simulink library "AEMS_Standard_Library"  (R2016b)
(part 7 of 39)

      |         maskobj_param(3).Enabled = 'on';
      |         switch(Outputs_From_get_param)
      |             case '1'
      |                 Non=4;
      |             case '2'
      |                 Non=5;
      |             case '3'
      |                 Non=6;
      |              case '4'
      |                  Non=7;
      |              case '6'
      |                  Non=9;
      |              case '8'
      |                  Non=11;
      |         end
      |     else
      |         maskobj_param(3).Visible = 'off';
      |         maskobj_param(3).Enabled = 'off';
      |         Non=4;
      |     end
      | for i=4:Non
      |     maskobj_param(i).Visible = 'on';
      |     maskobj_param(i).Enabled = 'on';
      | end
      | for i=Non+1:11
      |     maskobj_param(i).Visible = 'off';
      |     maskobj_param(i).Enabled = 'off';
      | end
      | clear maskobj_param;
      | clear maskobj;
      mask TypeOptions Dim_num: 1 | 2 | 3 | 4 | 6 | 8
      mask Callback Dim_num:
      | Outputs_From_get_param = get_param(gcb,'Dim_num');
      | Specificchoice_get_param = get_param(gcb,'Specificchoix');
      | maskobj = Simulink.Mask.get(gcbh);
      | maskobj_param = maskobj.Parameters;
      |     if strcmpi(Specificchoice_get_param,'on')
      |        Non=4;
      |         maskobj_param(3).Visible = 'on';
      |         maskobj_param(3).Enabled = 'on';
      |         switch(Outputs_From_get_param)
      |             case '1'
      |                 Non=4;
      |             case '2'
      |                 Non=5;
      |             case '3'
      |                 Non=6;
      |              case '4'
      |                  Non=7;
      |              case '6'
      |                  Non=9;
      |              case '8'
      |                  Non=11;
      |         end
      |     else
      |         maskobj_param(3).Visible = 'off';
      |         maskobj_param(3).Enabled = 'off';
      |         Non=4;
      |     end
      | for i=4:Non
      |     maskobj_param(i).Visible = 'on';
      |     maskobj_param(i).Enabled = 'on';
      | end
      | for i=Non+1:11
      |     maskobj_param(i).Visible = 'off';
      |     maskobj_param(i).Enabled = 'off';
      | end
      | clear maskobj_param;
      | clear maskobj;
      mask TypeOptions DemDebounceBehavior1: DEM_DEBOUNCE_FREEZE (0) | DEM_DEBOUNCE_RESET (1)
      mask TypeOptions DemDebounceBehavior2: DEM_DEBOUNCE_FREEZE (0) | DEM_DEBOUNCE_RESET (1)
      mask TypeOptions DemDebounceBehavior3: DEM_DEBOUNCE_FREEZE (0) | DEM_DEBOUNCE_RESET (1)
      mask TypeOptions DemDebounceBehavior4: DEM_DEBOUNCE_FREEZE (0) | DEM_DEBOUNCE_RESET (1)
      mask TypeOptions DemDebounceBehavior5: DEM_DEBOUNCE_FREEZE (0) | DEM_DEBOUNCE_RESET (1)
      mask TypeOptions DemDebounceBehavior6: DEM_DEBOUNCE_FREEZE (0) | DEM_DEBOUNCE_RESET (1)
      mask TypeOptions DemDebounceBehavior7: DEM_DEBOUNCE_FREEZE (0) | DEM_DEBOUNCE_RESET (1)
      mask TypeOptions DemDebounceBehavior8: DEM_DEBOUNCE_FREEZE (0) | DEM_DEBOUNCE_RESET (1)
      mask TypeOptions sampletime: 0.001 | 0.002 | 0.004 | 0.01 | 0.02 | 0.1
  AEMS_DEM_TIME_BASED_DEBOUNCE_THRSHOLD_DYN : Subsystem  Tag=[LIB]  Description=This subsystem is interface for self diagnosis standard calculated from similar condition and NG judgment.  mask(AEMS_DEM_TIME_BASED_DEBOUNCE_THRSHOLD_DYN){eventid=Dem_EventId_Device_Faulttype, Specificchoix=off, Dim_num=1, DemDebounceBehavior1=DEM_DEBOUNCE_FREEZE (0), DemDebounceBehavior2=DEM_DEBOUNCE_RESET (1), DemDebounceBehavior3=DEM_DEBOUNCE_FREEZE (0), DemDebounceBehavior4=DEM_DEBOUNCE_FREEZE (0), DemDebounceBehavior5=DEM_DEBOUNCE_RESET (1), DemDebounceBehavior6=DEM_DEBOUNCE_RESET (1), DemDebounceBehavior7=DEM_DEBOUNCE_FREEZE (0), DemDebounceBehavior8=DEM_DEBOUNCE_FREEZE (0), DemTimeBypassFailure=Cbx_dem_byp_fail_Device_Faulttype, sampletime=0.01, ToDataStoreMemory=off}
      mask prompts: eventid "Identifier of a diagnostic event (EventId)"; Specificchoix "Specific case used only for Nissan cases"; Dim_num "Time_Based_Debounce_Dimension"; DemDebounceBehavior1 "Dem Debounce Behavior 1"; DemDebounceBehavior2 "Dem Debounce Behavior 2"; DemDebounceBehavior3 "Dem Debounce Behavior 3"; DemDebounceBehavior4 "Dem Debounce Behavior 4"; DemDebounceBehavior5 "Dem Debounce Behavior 5"; DemDebounceBehavior6 "Dem Debounce Behavior 6"; DemDebounceBehavior7 "Dem Debounce Behavior 7"; DemDebounceBehavior8 "Dem Debounce Behavior 8"; DemTimeBypassFailure "Dem Debounce Time Bypass Failure"; sampletime "Sample Time"; ToDataStoreMemory "Write Output To Data Store Memory"
      mask help:
      | It  transmit the status Failed or Passed to the DEM. Accordingly,
      | some bits of the UDS DTC status byte changes synchronously or
      | asynchronously according to the configuration.
      |
      | -INPUTS-
      | conditionfulfilled: specifies whether the storage condition assigned
      | to the StorageConditionId is fulfilled
      | prefailed: Monitor reports nonqualified test result pre-failed
      | prepassed: Monitor reports nonqualified test result pre-passed
      | ClearDataRequest:Clears the Data Request value
      | reseteventdebounce: Freeze or reset the internal debounce timer.
      | failedthreshold: Defines the time out duration for "Event Failed" qualification.
      | passedthreshold: Defines the time out duration for "Event Passed" qualification.
      |
      | -OUTPUTS-
      | debouncevalue_for_failed: Value of debounce when an event failed
      | debouncevalue_for_passed: Value of debounce when an event passed
      | failed: Diagnostic monitor reports an event failed
      | passed: Diagnostic monitor reports an event passed
      |
      | -PARAMETERS-
      | EventId: Internal identifier of a diagnostic event. 0 is not a valid value.
      | Debounce Behavior: The event debounce counter will be frozen or reset
      | (0 for FREEZE and 1 for RESET)
      mask init:
      | lib_path = gcb;
      | Current_Child_Lib_Path = find_system(lib_path,'LookUnderMasks','all','FollowLinks','on','Name','AEMS_DEM_TIME_BASED_DEBOUNCE_THRSHOLD_DYN_D');
      | Attribute_Format_String_Part1 = '%<MaskType>\n EventId : %<eventid> \n Specific case used only for Nissan cases = %<Specificchoix> ';
      | Attribute_Format_String_Part2 = '';
      | if strcmpi(Specificchoix,'off')
      |     Dim_num = '1';
      | else
      |     Attribute_Format_String_Part2 = '\n Time_Based_Debounce_Dimention = %<Dim_num> ';
      | end
      | dim_block = ['AEMS_DEM_TIME_BASED_DEBOUNCE_THRSHOLD_DYN_' Dim_num 'D'];
      | 
      | rep_block = ['AEMS_Standard_Library/SUB/',dim_block];
      | if ismember(get_param(Current_Child_Lib_Path,'MaskType'),{dim_block})
      | else
      |     replace_block(lib_path,'FollowLinks','on','Name','AEMS_DEM_TIME_BASED_DEBOUNCE_THRSHOLD_DYN_D',rep_block,'noprompt');
      | end
      | 
      | Attribute_Format_String_Part3='';
      | for i=1:str2num(Dim_num)
      |     Attribute_Format_String_Part3=[Attribute_Format_String_Part3,'\n Dem Debounce Behavior ',num2str(i),' = %<DemDebounceBehavior',num2str(i),'>'];
      |     set_param([Current_Child_Lib_Path{:}],['DemDebounceBehavior',num2str(i)],get_param(lib_path,['DemDebounceBehavior',num2str(i)]));
      | end
      | 
      | sampletime_tmp = get_param(lib_path,'sampletime');
      | DemTimeBypassFailure_tmp = get_param(lib_path,'DemTimeBypassFailure');
      | 
      | set_param([Current_Child_Lib_Path{:}],'eventid',eventid);
      | set_param([Current_Child_Lib_Path{:}],'Sample_Time',sampletime_tmp);
      | set_param([Current_Child_Lib_Path{:}],'DemTimeBypassFailure',DemTimeBypassFailure_tmp);
      | 
      | %If To DataStoreMemory is enabled...
      | if strcmpi(ToDataStoreMemory,'on') && isempty(find_system(lib_path,'LookUnderMasks','all','FollowLinks','on','Name','AEMS_SRFLIPFLOP'))
      |     add_block('AEMS_Standard_Library/FLAG/AEMS_SRFLIPFLOP',[lib_path,'/AEMS_SRFLIPFLOP'],'Position',[930 254 1015 376]);
      |     add_block('simulink/Signal Attributes/Data Type Conversion',[lib_path,'/Data Type Conversion'],'Position',[1060 303 1115 327],'ShowName','off')
      |     add_block('simulink/Signal Routing/Data Store Write',[lib_path,'/Data Store Write'],'Position',[1160 302 1385 328],'ShowName','off');
      |     add_line(lib_path,'AEMS_DEM_TIME_BASED_DEBOUNCE_THRSHOLD_DYN_D/3','AEMS_SRFLIPFLOP/1','AutoRouting','on');
      |     add_line(lib_path,'AEMS_DEM_TIME_BASED_DEBOUNCE_THRSHOLD_DYN_D/4','AEMS_SRFLIPFLOP/2','AutoRouting','on');
      |     add_line(lib_path,'AEMS_SRFLIPFLOP/1','Data Type Conversion/1');
      |     add_line(lib_path,'Data Type Conversion/1','Data Store Write/1');
      | elseif strcmpi(ToDataStoreMemory,'off') && ~isempty(find_system(lib_path,'LookUnderMasks','all','FollowLinks','on','Name','AEMS_SRFLIPFLOP'))
      |     delete_block([lib_path,'/AEMS_SRFLIPFLOP']);
      |     delete_block([lib_path,'/Data Type Conversion']);
      |     delete_block([lib_path,'/Data Store Write']);
      |     delete_line(find_system(lib_path,'FollowLinks','on','FindAll','on','LookUnderMasks','on','Type','line','Connected','off'));
      | end
      | 
      | if strcmpi(ToDataStoreMemory,'on')
      |     %Get Task Rate of this block.(As per AEMS arch, all the blks shall be
      |     %kept under the runnable. The Runnable name will ncontain the sample
      |     %time suffix. From where we can get it.
      |     model_type_pos = strsplit(lib_path,'/');%to split all the layer paths in order to get the runnable path
      |     runnable_path = [bdroot '/' model_type_pos{2}];%to get the runnable or AIPCALL path
      |     trg_port_name = get_param(find_system(runnable_path,'BlockType','TriggerPort'),'Name');%to get the function call trigger name
      |     TaskRate = '';%the raster suffix is stored in the parameter
      |     
      |     if ~isempty(trg_port_name)
      |         trg_port_name_spltd = strsplit(trg_port_name{1},'_');%splitting is done in order to get the raster and its type(Sched or Event)
      |         
      |         % checking for rasters of type Sched or Event especially occuring in
      |         % runnables
      |         if ~isempty(regexp(trg_port_name_spltd{1},'^Sched|^Event','once'))
      |             TaskRate = ['_' regexprep(trg_port_name_spltd{1},'Sched|Event','','once')];
      |             
      |             %checking if the raster is dcmcb and this is applicable only for
      |             %APICALL
      |         elseif ~isempty(regexp([trg_port_name_spltd{1} '_' trg_port_name_spltd{2} '_' ],'^DataServices_DCM_|^RoutineServices_DCM_','once'))||...
      |                 ~isempty(regexp(trg_port_name_spltd{1},'^Dcm$','once'))
      |             TaskRate = '_dcmcb';
      |             
      |             %checking if this block is used under the function call trigger
      |             %starting with "Com" and then giving an error message
      |             %this is applicable only for APICALL
      |         elseif ~isempty(regexp(trg_port_name_spltd{1},'^Com$','once'))
      |             msg = sprintf(['\n','The FIM block "' lib_path '" should not be present within APICALLs having function call trigger as "Com"']);
      |             errordlg(msg);
      |             return;
      |         end
      |     end
      |     DataStoreName = [eventid,TaskRate];
      |     set_param([lib_path,'/Data Store Write'],'DataStoreName',DataStoreName);
      | end
      | 
      | Attribute_Format_String_Part5 = '\n Write Output To Data Store Memory := %<ToDataStoreMemory>';
      | 
      | 
      | Attribute_Format_String_Part4='\nDem Debounce Time Bypass Failure = %<DemTimeBypassFailure>\nSample Time = %<sampletime>';
      | Attribute_Format_String = [Attribute_Format_String_Part1,Attribute_Format_String_Part2,Attribute_Format_String_Part3,Attribute_Format_String_Part4, Attribute_Format_String_Part5];
      | 
      | set_param(lib_path,'AttributesFormatString',Attribute_Format_String);
      settings: AttributesFormatString=%<MaskType>\n EventId : %<eventid> \n Specific case used only for Nissan cases = %<Specificchoix> \n Dem Debounce Behavior 1 = %<DemDebounceBehavior1>\nDem Debounce Time Bypass Failure = %<DemTimeBypassFailure>\nSample Time = %<sampletime>\n Write Output To Data Store Memory := %<ToDataStoreMemory>
      mask Help:
      | eval('path_lib=fileparts(which(''AEMS_Standard_Library''));');
      | doc_path = [path_lib '\help\AEMS_DEM_TIME_BASED_DEBOUNCE_THRSHOLD_DYN.pdf'];
      | eval('open(doc_path)');
      mask Callback eventid:
      | lib_path=gcb;
      | EventID=get_param(lib_path,'eventid');
      | Splitname=regexp(EventID,'_','all');
      | EventID_Name=extractAfter(EventID,EventID(1:Splitname(2)));
      | BypassFailure=strcat('Cbx_dem_byp_fail_',EventID_Name);
      | set_param(lib_path,'DemTimeBypassFailure',BypassFailure);
      | ToDataStoreMemory = get_param(lib_path,'ToDataStoreMemory');
      | 
      | if strcmpi(ToDataStoreMemory,'on')
      | model_type_pos = strsplit(lib_path,'/');%to split all the layer paths in order to get the runnable path
      | runnable_path = [bdroot '/' model_type_pos{2}];%to get the runnable or AIPCALL path
      | trg_port_name = get_param(find_system(runnable_path,'BlockType','TriggerPort'),'Name');%to get the function call trigger name
      | TaskRate = '';%the raster suffix is stored in the parameter
      | 
      | if ~isempty(trg_port_name)
      |     trg_port_name_spltd = strsplit(trg_port_name{1},'_');%splitting is done in order to get the raster and its type(Sched or Event)
      | 
      |     % checking for rasters of type Sched or Event especially occuring in
      |     % runnables
      |     if ~isempty(regexp(trg_port_name_spltd{1},'^Sched\d+(ms|s)$|^Event+(sync|knock|comc|coml|dcmcb)$','once'))
      |         TaskRate = ['_' regexp(trg_port_name_spltd{1},'\d+(ms|s)$|sync$|knock$|comc$|coml$|dcmcb$','match','once')];
      | 
      |     %checking if the raster is dcmcb and this is applicable only for
      |     %APICALL
      |     elseif ~isempty(regexp([trg_port_name_spltd{1} '_' trg_port_name_spltd{2} '_' ],'^DataServices_DCM_|^RoutineServices_DCM_','once'))||...
      |             ~isempty(regexp(trg_port_name_spltd{1},'^Dcm$','once'))
      |         TaskRate = '_dcmcb';
      | 
      |     %checking if this block is used under the function call trigger
      |     %starting with "Com" and then giving an error message
      |     %this is applicable only for APICALL
      |     elseif ~isempty(regexp(trg_port_name_spltd{1},'^Com$','once'))
      |         msg = sprintf(['\n','The DEM blocks "' Thisblk '" should not be present within APICALLs having function call trigger as "Com"']);
      |         errordlg(msg);
      |         return;
      |     end
      | end
      | DataStoreName = [EventID TaskRate];%the variable name that should be given to DataStoreRead block
      | set_param([lib_path,'/Data Store Write'],'DataStoreName',DataStoreName);
      | else
      |     %do nothing
      | end
      mask Callback Specificchoix:
      | Outputs_From_get_param = get_param(gcb,'Dim_num');
      | Specificchoice_get_param = get_param(gcb,'Specificchoix');
      | maskobj = Simulink.Mask.get(gcbh);
      | maskobj_param = maskobj.Parameters;
      |     if strcmpi(Specificchoice_get_param,'on')
      |        Non=4;
      |         maskobj_param(3).Visible = 'on';
      |         maskobj_param(3).Enabled = 'on';
      |         switch(Outputs_From_get_param)
      |             case '1'
      |                 Non=4;
      |             case '2'
      |                 Non=5;
      |             case '3'
      |                 Non=6;
      |              case '4'
      |                  Non=7;
      |              case '6'
      |                  Non=9;
      |              case '8'
      |                  Non=11;
      |         end
      |     else
      |         maskobj_param(3).Visible = 'off';
      |         maskobj_param(3).Enabled = 'off';
      |         Non=4;
      |     end
      | for i=4:Non
      |     maskobj_param(i).Visible = 'on';
      |     maskobj_param(i).Enabled = 'on';
      | end
      | for i=Non+1:11
      |     maskobj_param(i).Visible = 'off';
      |     maskobj_param(i).Enabled = 'off';
      | end
      | clear maskobj_param;
      | clear maskobj;
      mask TypeOptions Dim_num: 1 | 2 | 3 | 4 | 6 | 8
      mask Callback Dim_num:
      | Outputs_From_get_param = get_param(gcb,'Dim_num');
      | Specificchoice_get_param = get_param(gcb,'Specificchoix');
      | maskobj = Simulink.Mask.get(gcbh);
      | maskobj_param = maskobj.Parameters;
      |     if strcmpi(Specificchoice_get_param,'on')
      |        Non=4;
      |         maskobj_param(3).Visible = 'on';
      |         maskobj_param(3).Enabled = 'on';
      |         switch(Outputs_From_get_param)
      |             case '1'
      |                 Non=4;
      |             case '2'
      |                 Non=5;
      |             case '3'
      |                 Non=6;
      |              case '4'
      |                  Non=7;
      |              case '6'
      |                  Non=9;
      |              case '8'
      |                  Non=11;
      |         end
      |     else
      |         maskobj_param(3).Visible = 'off';
      |         maskobj_param(3).Enabled = 'off';
      |         Non=4;
      |     end
      | for i=4:Non
      |     maskobj_param(i).Visible = 'on';
      |     maskobj_param(i).Enabled = 'on';
      | end
      | for i=Non+1:11
      |     maskobj_param(i).Visible = 'off';
      |     maskobj_param(i).Enabled = 'off';
      | end
      | clear maskobj_param;
      | clear maskobj;
      mask TypeOptions DemDebounceBehavior1: DEM_DEBOUNCE_FREEZE (0) | DEM_DEBOUNCE_RESET (1)
      mask TypeOptions DemDebounceBehavior2: DEM_DEBOUNCE_FREEZE (0) | DEM_DEBOUNCE_RESET (1)
      mask TypeOptions DemDebounceBehavior3: DEM_DEBOUNCE_FREEZE (0) | DEM_DEBOUNCE_RESET (1)
      mask TypeOptions DemDebounceBehavior4: DEM_DEBOUNCE_FREEZE (0) | DEM_DEBOUNCE_RESET (1)
      mask TypeOptions DemDebounceBehavior5: DEM_DEBOUNCE_FREEZE (0) | DEM_DEBOUNCE_RESET (1)
      mask TypeOptions DemDebounceBehavior6: DEM_DEBOUNCE_FREEZE (0) | DEM_DEBOUNCE_RESET (1)
      mask TypeOptions DemDebounceBehavior7: DEM_DEBOUNCE_FREEZE (0) | DEM_DEBOUNCE_RESET (1)
      mask TypeOptions DemDebounceBehavior8: DEM_DEBOUNCE_FREEZE (0) | DEM_DEBOUNCE_RESET (1)
      mask TypeOptions sampletime: 0.001 | 0.002 | 0.004 | 0.01 | 0.02 | 0.1
  AEMS_FIM_GETFUNCTIONINHIBITION : Subsystem  Tag=[LIB]  mask(AEMS_FIM_GETFUNCTIONINHIBITION){FIDshortName=Fim_fid_xxxx, Specificchoix=off, Dim_num=1, FunctionMode=Functional}
      mask prompts: FIDshortName "Downgraded mode name :"; Specificchoix "Specific case used only for Nissan cases"; Dim_num "Dimension :"; FunctionMode "Function Mode"
      mask help:
      | [Get Function Permission]
      | - Refer the AUTOSAR FiM_GetFunctionPermission [SWS_Fim_00011]
      |
      | -OUTPUTS-
      | InhibitionStatus: Inhibition status
      |
      | -PARAMETERS-
      | Downgraded mode name : Enter downgraded mode name according to AEMS naming rules
      mask init:
      | % FID = ['Fim_FID_' FIDshortName];
      | % eval([char(FID) '= 0;'])
      | lib_path = gcb;
      | if strcmpi(Specificchoix,'off')
      |    Dim_num='1'; 
      | end
      | %Specify child
      | % child_lib = find_system(lib_path,'LookUnderMasks','all','FollowLinks','on','Name','AEMS_FIM_GET_FUNC_PMT_D');
      | child_lib = {[lib_path,'/AEMS_FIM_GET_FUNC_PMT_D']};
      | 
      | switch Dim_num
      |     case '1'
      |         if ismember(get_param(child_lib,'MaskType'),{'AEMS_FIM_GET_FUNC_PMT_1D'})
      |         else
      |             replace_block(lib_path,'FollowLinks','on','Name','AEMS_FIM_GET_FUNC_PMT_D','AEMS_Standard_Library/SUB/AEMS_FIM_GET_FUNC_PMT_1D','noprompt');
      |         end
      |     case '2'
      |         if ismember(get_param(child_lib,'MaskType'),{'AEMS_FIM_GET_FUNC_PMT_2D'})
      |         else
      |             replace_block(lib_path,'FollowLinks','on','Name','AEMS_FIM_GET_FUNC_PMT_D','AEMS_Standard_Library/SUB/AEMS_FIM_GET_FUNC_PMT_2D','noprompt');
      |         end
      | end
      | 
      | %Set parameters
      | % set_param([child_lib{:}],'FIDshortName',char(FIDshortName));
      | set_param([child_lib{:}],'FID',char(FIDshortName));
      | set_param([child_lib{:}],'FunctionMode',FunctionMode);
      settings: AttributesFormatString=%<MaskType>\nDowngraded mode name : = %<FIDshortName>\nSpecific case used only for Nissan cases = %<Specificchoix>\nFunction Mode = %<FunctionMode>
      mask Help:
      | eval('path_lib=fileparts(which(''AEMS_Standard_Library''));');
      | mskblk=get_param(gcbh,'MaskType');
      | doc_path = [path_lib '\Help\',mskblk,'.pdf'];
      | eval('open(doc_path)');
      mask Callback Specificchoix:
      | maskobj = Simulink.Mask.get(gcbh);
      | maskobj_param = maskobj.Parameters;
      | 
      | if strcmp(get(gcbh,'Specificchoix'),'on')
      |     maskobj_param(3).Visible = 'on';
      |     maskobj_param(3).Enabled = 'on';
      | else
      |     maskobj_param(3).Visible = 'off';
      |     maskobj_param(3).Enabled = 'off';
      | end
      | clear maskobj_param;
      | clear maskobj;
      mask TypeOptions Dim_num: 1 | 2
      mask TypeOptions FunctionMode: Functional | Dysfunctional | From Data Store memory
      mask Display:
      | dgn_mask = ['Downgraded mode name \n ' FIDshortName];
      | 
      | if strcmpi(Specificchoix,'on')
      |     set(gcbh,'AttributesFormatString','%<MaskType>\nDowngraded mode name : = %<FIDshortName>\nSpecific case used only for Nissan cases = %<Specificchoix>\nDimension : = %<Dim_num>\nFunction Mode = %<FunctionMode>');
      | else
      |     set(gcbh,'AttributesFormatString','%<MaskType>\nDowngraded mode name : = %<FIDshortName>\nSpecific case used only for Nissan cases = %<Specificchoix>\nFunction Mode = %<FunctionMode>');
      | end
      | 
      | disp(dgn_mask);
      | plot([5,5,5])
      | plot([6,6,6])
